simulink model "PI_vectorial"  (R2021b)
settings: Solver=VariableStepAuto  StartTime=0.0  StopTime=10.0  RelTol=1e-3
undefined symbols (not defined in the file): K, ki
libraries: arduinolib x2
settings Model: Creator=parra  LastModifiedBy=parra

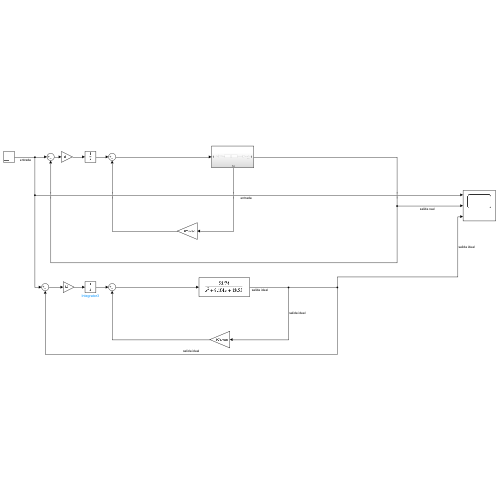
[thumbnail: Simulink's stored preview of the top-level diagram]
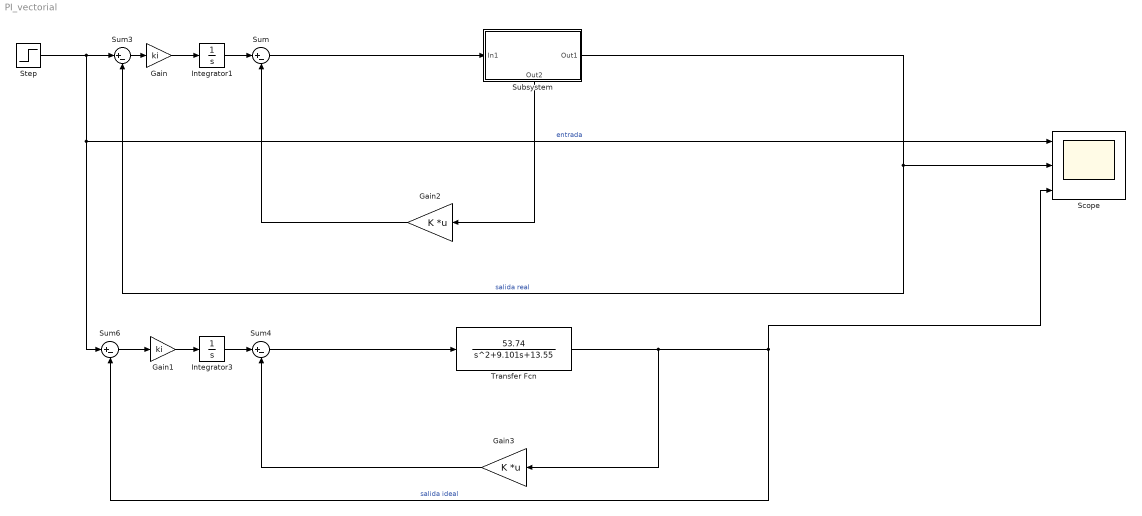
== system PI_vectorial ==
  Gain : Gain  Gain=ki
  Gain1 : Gain  Gain=ki
  Gain2 : Gain  Gain=K  Multiplication=Matrix(K*u) (u vector)
  Gain3 : Gain  Gain=K  Multiplication=Matrix(K*u) (u vector)
  Integrator1 : Integrator
  Integrator3 : Integrator
  Scope : Scope  NumInputPorts=3
  Step : Step  Time=20  Before=0.5  SampleTime=0.01
  Subsystem : Subsystem
      settings: PortSchema="{\"entries\":[{\"content\":{\"sides\":[{\"content\":{\"connectorIds\":[\"In1\"]},\"type\":\"ConnectorPlacement.EquallySpacedRectSide\",\"uuid\":\"022f3360-9ec3-4b89-a239-897e1b8bdd20\"},{\"content\":{\"connectorIds\":[\"Out1\"],\"side\":\"RIGHT\"},\"type\":\"ConnectorPlacement.EquallySpacedRectSide\",\"uuid\":\"6de92038-29b0-4288-99b7-2cb051fb1c3f\"},{\"content\":{\"side\":\"TOP\"},\"type\":\"ConnectorPlacement.EquallySpacedRectSide\",\"uuid\":\"ed85708b-cbc2-40d6-ba3b-fc5403f14d68\"},{\"content\":{\"connectorIds\":[\"Out2\"],\"side\":\"BOTTOM\"},\"type\":\"ConnectorPlacement.EquallySpacedRectSide\",\"uuid\":\"1f485459-5873-46b6-8d75-9d4b5ba46813\"}]},\"type\":\"ConnectorPlacement.EquallySpacedConnector\",\"uuid\":\"05ff1f01-a647-4d8b-bf50-9915a134f63a\"}],\"packageUris\":[\"http://schema.mathworks.com/mf0/Connector/R2020b\"],\"version\":\"1.0\"}"
  Sum{,3..4,6} (4 alike) : Sum  Inputs=|+-
  Transfer Fcn : TransferFcn  Numerator=[53.74]  Denominator=[1 9.101 13.55]
  wires:
  Step/1 -> Sum3/1, Sum6/1, Scope/1  "entrada"
  Gain2/1 -> Sum/2
  Sum/1 -> Subsystem/1(In1)
  Sum3/1 -> Gain/1
  Integrator1/1 -> Sum/1
  Gain/1 -> Integrator1/1
  Subsystem/1(Out1) -> Sum3/2, Scope/2  "salida real"
  Subsystem/2(Out2) -> Gain2/1
  Transfer Fcn/1 -> Gain3/1, Scope/3, Sum6/2  "salida ideal"
  Sum4/1 -> Transfer Fcn/1
  Gain3/1 -> Sum4/2
  Integrator3/1 -> Sum4/1
  Gain1/1 -> Integrator3/1
  Sum6/1 -> Gain1/1

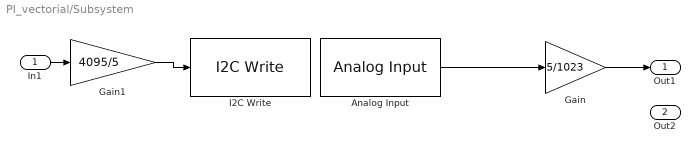
== system PI_vectorial/Subsystem ==
  In1 : Inport
  Analog Input : arduinolib/Analog Input  pinNumber=1  ReadResultsOnly=off  ConversionTriggerSource=Software  ExternalTriggerType=uint32( 0 )  OutputDataType=uint16  EnableConversionCompleteNotify=off  EnableOuputStatus=off  SampleTime=0.01  blockPlatform=arduino
  Gain : Gain  Gain=5/1023
  Gain1 : Gain  Gain=4095/5  OutDataTypeStr=uint16
  I2C Write : arduinolib/I2C Write  I2CModule=0  Mode=Master  SlaveAddress=96  SlaveByteOrder=BigEndian  Direction=Transmitter  RegisterAddressMode=off  RegisterAddress=0  SlaveDataType=uint8  DataLength=1  NoAck=off  RepeatedStart=off  OutputStatus=off  blockPlatform=ARDUINO
      settings: SourceProductBaseCode=ARDUINO
  Out1 : Outport
  Out2 : Outport  Port=2
  wires:
  Gain1/1 -> I2C Write/1
  In1/1 -> Gain1/1
  Gain/1 -> Out1/1
  Analog Input/1 -> Gain/1
